simulink model "sl_groundvehicleDynamicsV1"  (R2020b)
settings: Solver=ode45  StartTime=0.0  StopTime=4000  RelTol=1e-5  EnableMultiTasking=on
InitFcn:
  | load('sim_parameters')
values from neighbouring files (symbols this model uses):
  dt = 0.01    [sim_parameters.mat]
  mot_B =     [sim_parameters.mat]
  mot_COM =     [sim_parameters.mat]
  pp_cont =     [sim_parameters.mat]
  Ts = block.DialogPrm(1).Data    [bh_ddr_animate_sfun.m]    (also in sim_parameters.mat = 0.01)
  veh =     [sim_parameters.mat]
undefined symbols (not defined in the file or in its folder): DiscIntNeverNeededParam, Ke, obstacles, waypoints
libraries: pid_lib x4, mobileRoboticsLib x3, simulink_extras x3, simulink x1
(part 2 of 2)

== matlab function sl_groundvehicleDynamicsV1/Path Planning ==
  data: wpt_tolerance input; state input; pathVector output; waypoints input; s output; avgCapErr output
function [pathVector,s, avgCapErr] = fcn(wpt_tolerance, state, waypoints)

%initalise stop trigger
s = 0;
%initalise average capture error
avgCapErr = 0;

%persistent variables;
persistent index;
persistent vector;
persistent captureError;

% initialise persistent variables when empty
if isempty(index)
    index = 1;
end
if isempty(vector)
     vector = zeros(2,100);
end
if isempty(captureError)
    captureError = 1000.*ones(1,length(waypoints));
end


%vehicle state
x = state(1);
y = state(2);

%desired location
DWP = zeros(1,2);
DWP(1) = waypoints(index,1);
DWP(2) = waypoints(index,2);

%past location
PWP = pastWaypoint(waypoints, index);

%optimal path vector
%if the vector for this waypoint has been computed it won't recompute
if ~any(vector, 'all')
    vector = createVector();
end

pathVector = vector;

%distance and to target waypoint
dist = calcDist(DWP);

%distance and to past waypoint
pastDist = calcDist(PWP);

% if within the capture tolerence see if we are at the closest point
if pastDist < wpt_tolerance && index > 1
    if pastDist < captureError(index-1)
        captureError(index-1) = pastDist;
    end
end 
    
%if at final waypoint
if dist < wpt_tolerance && index == length(waypoints)

    %set capture error to threshold
    captureError(length(captureError)) = wpt_tolerance;

    %calculate avg capture error
    avgCapErr = mean(captureError);

    % stop simulation
    s = 1; 

%if at current desired waypoint
elseif dist < wpt_tolerance
     index = index+1;
     %calculate new path vector for next WP
     vector = zeros(2,100);
end
 
%%%%%%%%%Additional functions%%%%%%%%%%%%%%%

%%function to get the past way point coordinates
    function [PWP] = pastWaypoint(waypoints, index)
        PWP = zeros(1,2);
        x_init = 2; % initial x and y pos of robot
        y_init = 2;
        
        %this should make it go direcly to the first WP or will set
        %the last waypoint as the previous WP if past the first WP
        if (index == 1)
            PWP(1) = x_init;
            PWP(2) = y_init; 
        else
            PWP(1) = waypoints(index-1,1);
            PWP(2) = waypoints(index-1,2);
        end
    end

%%function to make vector between old and new waypoint
    function [vector] = createVector()
        stepNum = 100;
        
        %creates a vector of the x points and calculated y points for those
        %points
        vectorX = linspace(PWP(1),DWP(1),stepNum);
        
        %check if waypoints have same x coord
        if PWP(1) == DWP(1)
            vectorY = linspace(PWP(2),DWP(2),stepNum);
        else %interpolate normally
            vectorY = interp1([PWP(1),DWP(1)],[PWP(2),DWP(2)],vectorX);
        end        
        
        %concatenates vectors
        vector = zeros(2,100);%length(vectorX));
        vector(1,:) = vectorX;
        vector(2,:) = vectorY;
    end

%%function to calulate the stright line distance between curent pos and 
%%specified point
    function [dist] = calcDist(point)
        dx = point(1) - x;
        dy = point(2) - y;
        dist = sqrt(dx^2 + dy^2);
    end

end

== matlab function sl_groundvehicleDynamicsV1/Controller/Turn Rate Controller/Turn Rate Limiter ==
  data: error input; psi_star output
function psi_star = fcn(error)
    % determine direction of robot, and turn by constant amount until
    % within guidance angle
    turn_rate = deg2rad(180);
    psi_star = sign(error)*turn_rate;

== matlab function sl_groundvehicleDynamicsV1/Controller/Velocity Controller ==
  data: error input; v_star output
function v_star = fcn(error)
    % proportional control
    max_speed = 1.3; % m/s (breaks at higher than 1.3)
    % want to reach max speed when within 30 degrees of target
    angle_thresh = deg2rad(30);
    gain = max_speed/(1 - angle_thresh/pi);
    % calculate the relative speed
    v_star = gain * (1 - abs(error/pi));
    if v_star > max_speed
        v_star = max_speed;
    end
